simulink model "TugasElin"  (R2021a)
settings: Solver=VariableStepAuto  StartTime=0.0  StopTime=10.0  RelTol=1e-3
settings Model: Creator=asus  LastModifiedBy=asus

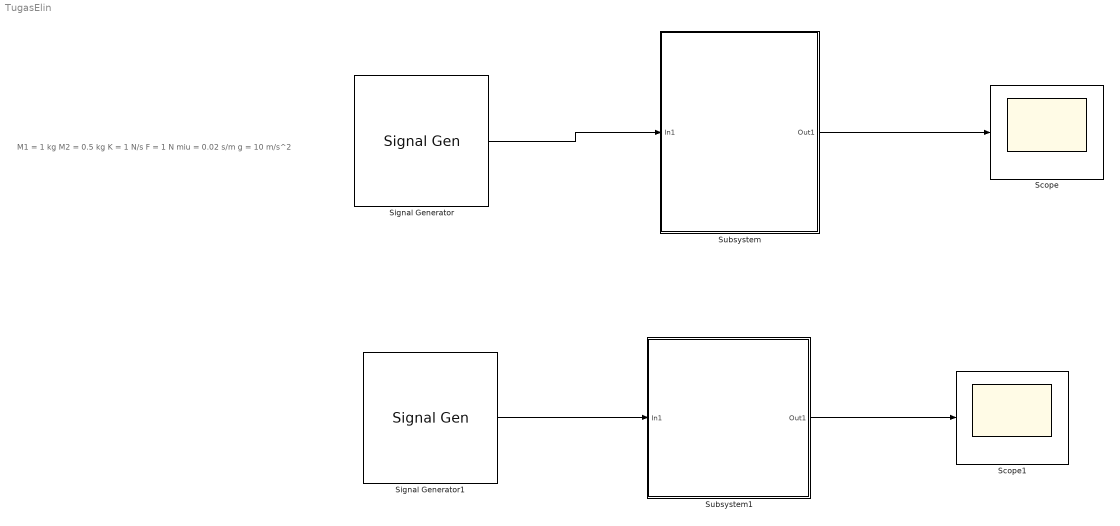
== system TugasElin ==
  note: M1 = 1 kg
      | M2 = 0.5 kg
      | K = 1 N/s
      | F = 1 N
      | miu = 0.02 s/m
      | g = 10 m/s^2
  Scope : Scope
  Scope1 : Scope
  Signal Generator : SignalGenerator  WaveForm=square  Amplitude=-1  Frequency=0.001
  Signal Generator1 : SignalGenerator  WaveForm=square  Units=rad/sec
  Subsystem : Subsystem  mask(Train System){Mk=0.02, M1=1, g=10, x1=56.4, x2=60, k=1}
      mask help: Silakan ubah nilai berikut
      mask init:
      | Mk > 0
      | M1 > 0
      | g > 0
      | x1 > 0
      | x2 > 0
      | k > 0
      mask Display: image("C:\Users\asus\Downloads\pngtree-cartoon-train-illustration-png-image_8780793.png")
  Subsystem1 : Subsystem  mask(Car Spot){k=1, x1=3, M2=0.5, Miu=0.02, g=10, x2=4}
      mask help: Silakan mengubah nilai parameter berikut
      mask init:
      | k > 0
      | x1 > 0
      | x2 > 0
      | M2 > 0
      | g > 0
      | Miu > 0
      mask Display: image("C:\Users\asus\Downloads\images.jpeg")
  wires:
  Subsystem/1(Out1) -> Scope/1
  Subsystem1/1(Out1) -> Scope1/1
  Signal Generator1/1 -> Subsystem1/1(In1)
  Signal Generator/1 -> Subsystem/1(In1)

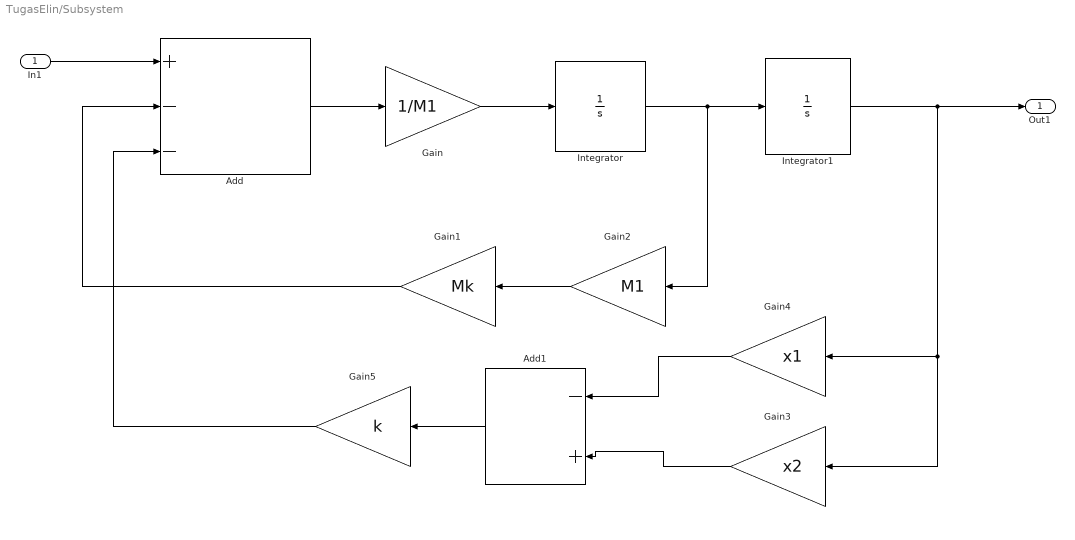
== system TugasElin/Subsystem ==
  In1 : Inport
  Add : Sum  Inputs=+--
  Add1 : Sum  Inputs=-+
  Gain : Gain  Gain=1/M1
  Gain1 : Gain  Gain=Mk
  Gain2 : Gain  Gain=M1
  Gain3 : Gain  Gain=x2
  Gain4 : Gain  Gain=x1
  Gain5 : Gain  Gain=k
  Integrator : Integrator
  Integrator1 : Integrator
  Out1 : Outport
  wires:
  In1/1 -> Add/1
  Add/1 -> Gain/1
  Gain/1 -> Integrator/1
  Integrator/1 -> Gain2/1, Integrator1/1
  Gain2/1 -> Gain1/1
  Gain1/1 -> Add/2
  Integrator1/1 -> Gain3/1, Gain4/1, Out1/1
  Gain4/1 -> Add1/1
  Gain3/1 -> Add1/2
  Add1/1 -> Gain5/1
  Gain5/1 -> Add/3

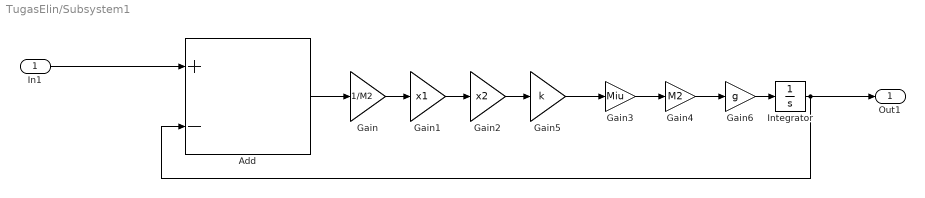
== system TugasElin/Subsystem1 ==
  In1 : Inport
  Add : Sum  Inputs=+-
  Gain : Gain  Gain=1/M2
  Gain1 : Gain  Gain=x1
  Gain2 : Gain  Gain=x2
  Gain3 : Gain  Gain=Miu
  Gain4 : Gain  Gain=M2
  Gain5 : Gain  Gain=k
  Gain6 : Gain  Gain=g
  Integrator : Integrator
  Out1 : Outport
  wires:
  Gain5/1 -> Gain3/1
  Gain3/1 -> Gain4/1
  Add/1 -> Gain/1
  In1/1 -> Add/1
  Gain6/1 -> Integrator/1
  Gain4/1 -> Gain6/1
  Integrator/1 -> Add/2, Out1/1
  Gain/1 -> Gain1/1
  Gain1/1 -> Gain2/1
  Gain2/1 -> Gain5/1
